simulink library "cst"  (Simulink 8.1)
settings: Solver=ode1  StartTime=0.0  StopTime=Inf  FixedStep=0.001  RelTol=1e-3
PostLoadFcn:
  | , if any(exist('dsrtsu_mdlpostloadfcn', 'file') == [2, 3, 6]), try dsrtsu_mdlpostloadfcn('Execute', bdroot); catch fprintf('Error in PostLoadFcn (dsrtsu_mdlpostloadfcn) for model "%s":\n %s\n', bdroot, lasterr); end, end,
undefined symbols (not defined in the file or in its folder): FALSE, KJUD_ACCSpdMErrorGParam_num, KJUD_ACCSpdMFFParam_num, KJUD_ACCSpdMInitialIParam_num, KJUD_ACCSpdMKdParam_num, KJUD_ACCSpdMKiParam_num, KJUD_ACCSpdMKpParam_num, KJUD_ACCSpdMMaxIParam_num, KJUD_ACCSpdMMinIParam_num, KJUD_ACCSpdMResetIParam_num
libraries: hcu_lib x1
settings Model: DSRTSU_INTERNAL_RTI_VER=450  DSRTSU_INTERNAL_RTI_TYPE=rti1401  RTICANMMDATA=struct('GeneralSetupData',struct('modelroot','D:\Projects\ELN150201\Repositories\Taiwan\trunk\AdasDragon\software\sw_development\arch\app\jud','generalsettings',struct('filesettings',struct('destfolder',struct('Name','RTICANMM_FILES','Check',1),'buildfolder',struct('Name','.','Check',1),'AbsDestfolder',struct('Name','D:\Projects\ELN150201\Repositories\Taiwan\trunk\AdasDragon\software\sw_development\arch\app\jud\RTICANMM_FILES'),'AbsBuildfolder',struct('Name','D:\Projects\ELN150201\Repositories\Taiwan\trunk\AdasDragon\software\sw_development\arch\app\jud'))),'options',struct('addpaths',1,'rmpaths',1,'addtrcexclusion',logical(1),'cannavigator',struct('checkmonitoring',0),'show_usrtrc',0,'use_usrtrc',0),'advanced',struct('options',[1 1 1 1 1 1 1 1 1 1 1 1 1 1 1 1 1 1 1 1 1 1 1 1 1 1 1 1 1 1 1 1 1 1 1 1 1 1 1 1 1 1 1 1 1 1 1 1 1 1 1 1 1 1 1 1 1 1 1 1 1 1 1 1 1 1 1 1 1 1 1 1 1 1 1 1 1 1 1 1 1 1 1 1 1 1 1 1 1 1 1 1 1 1 1 1 1 1 1 1]),'MPSetup',{{}},'modelname','cst','block','cst'))  DSRTSU_INTERNAL_RTIFPGA=40  Creator=AT015411  LastModifiedBy=AT015086

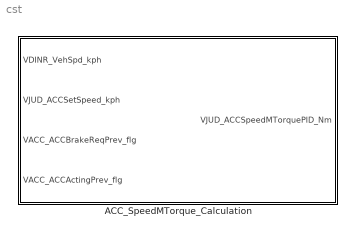
== system cst ==
  ACC_SpeedMTorque_Calculation : Subsystem

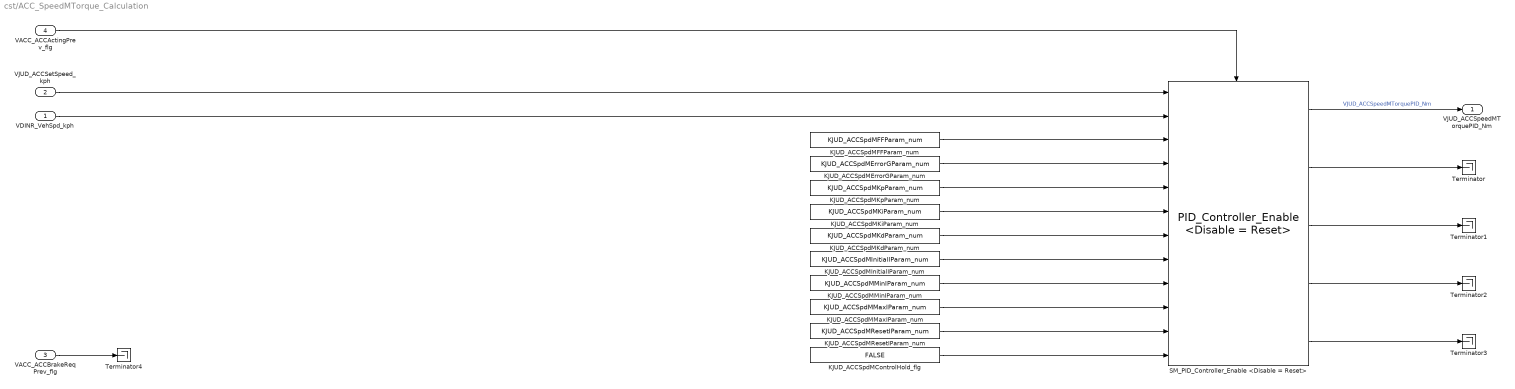
== system cst/ACC_SpeedMTorque_Calculation ==
  VDINR_VehSpd_kph : Inport
  VJUD_ACCSetSpeed_kph : Inport  Port=2
  VACC_ACCBrakeReqPrev_flg : Inport  Port=3
  VACC_ACCActingPrev_flg : Inport  Port=4
  KJUD_ACCSpdMControlHold_flg : Constant  Value=FALSE  OutDataTypeStr=boolean
  KJUD_ACCSpdMErrorGParam_num : Constant  Value=KJUD_ACCSpdMErrorGParam_num
  KJUD_ACCSpdMFFParam_num : Constant  Value=KJUD_ACCSpdMFFParam_num
  KJUD_ACCSpdMInitialIParam_num : Constant  Value=KJUD_ACCSpdMInitialIParam_num
  KJUD_ACCSpdMKdParam_num : Constant  Value=KJUD_ACCSpdMKdParam_num
  KJUD_ACCSpdMKiParam_num : Constant  Value=KJUD_ACCSpdMKiParam_num
  KJUD_ACCSpdMKpParam_num : Constant  Value=KJUD_ACCSpdMKpParam_num
  KJUD_ACCSpdMMaxIParam_num : Constant  Value=KJUD_ACCSpdMMaxIParam_num
  KJUD_ACCSpdMMinIParam_num : Constant  Value=KJUD_ACCSpdMMinIParam_num
  KJUD_ACCSpdMResetIParam_num : Constant  Value=KJUD_ACCSpdMResetIParam_num
  SM_PID_Controller_Enable <Disable = Reset> : hcu_lib/PID_Controller_Enable <Disable = Reset>  SystemSampleTime=-1
  Terminator{,1..4} (5 alike) : Terminator
  VJUD_ACCSpeedMTorquePID_Nm : Outport
  wires:
  VDINR_VehSpd_kph/1 -> SM_PID_Controller_Enable <Disable = Reset>/2
  VJUD_ACCSetSpeed_kph/1 -> SM_PID_Controller_Enable <Disable = Reset>/1
  SM_PID_Controller_Enable <Disable = Reset>/1 -> VJUD_ACCSpeedMTorquePID_Nm/1  "VJUD_ACCSpeedMTorquePID_Nm"
  KJUD_ACCSpdMKiParam_num/1 -> SM_PID_Controller_Enable <Disable = Reset>/6
  KJUD_ACCSpdMInitialIParam_num/1 -> SM_PID_Controller_Enable <Disable = Reset>/8
  KJUD_ACCSpdMMinIParam_num/1 -> SM_PID_Controller_Enable <Disable = Reset>/9
  KJUD_ACCSpdMMaxIParam_num/1 -> SM_PID_Controller_Enable <Disable = Reset>/10
  KJUD_ACCSpdMResetIParam_num/1 -> SM_PID_Controller_Enable <Disable = Reset>/11
  KJUD_ACCSpdMFFParam_num/1 -> SM_PID_Controller_Enable <Disable = Reset>/3
  KJUD_ACCSpdMErrorGParam_num/1 -> SM_PID_Controller_Enable <Disable = Reset>/4
  VACC_ACCActingPrev_flg/1 -> SM_PID_Controller_Enable <Disable = Reset>/Enable
  SM_PID_Controller_Enable <Disable = Reset>/2 -> Terminator/1
  SM_PID_Controller_Enable <Disable = Reset>/3 -> Terminator1/1
  SM_PID_Controller_Enable <Disable = Reset>/4 -> Terminator2/1
  SM_PID_Controller_Enable <Disable = Reset>/5 -> Terminator3/1
  KJUD_ACCSpdMControlHold_flg/1 -> SM_PID_Controller_Enable <Disable = Reset>/12
  KJUD_ACCSpdMKpParam_num/1 -> SM_PID_Controller_Enable <Disable = Reset>/5
  KJUD_ACCSpdMKdParam_num/1 -> SM_PID_Controller_Enable <Disable = Reset>/7
  VACC_ACCBrakeReqPrev_flg/1 -> Terminator4/1
